simulink model "mainmodel"  (R2020a)
settings: Solver=VariableStepAuto  StartTime=0.0  StopTime=10.0  MaxStep=0.04  RelTol=1e-3
undefined symbols (not defined in the file): Iei, Iv, Rfd, Rw
settings Model: Creator=Bhanu  LastModifiedBy=Bhanu

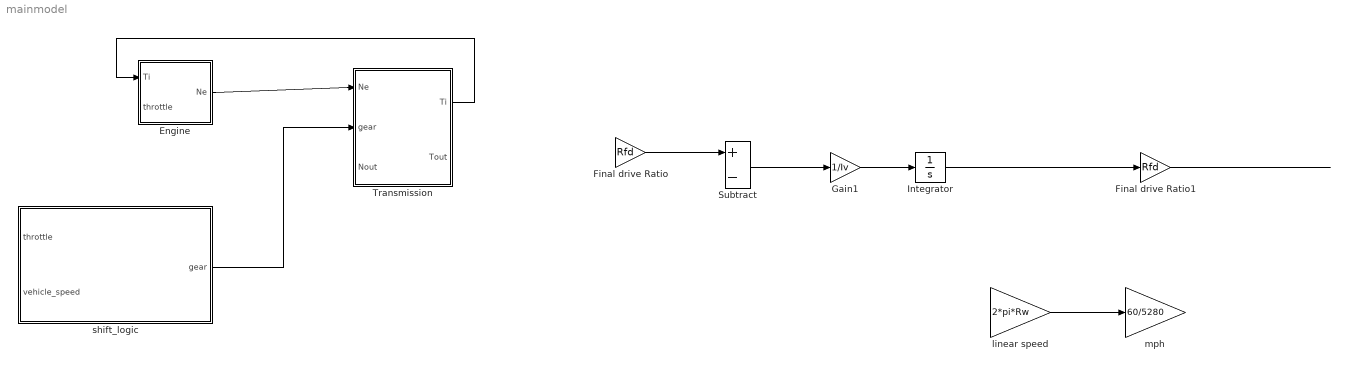
== system mainmodel ==
  "Engine " : Subsystem
  Final drive Ratio : Gain  Gain=Rfd
  Final drive Ratio1 : Gain  Gain=Rfd
  Gain1 : Gain  Gain=1/Iv
  Integrator : Integrator
  Subtract : Sum  Inputs=+-
  "Transmission " : Subsystem
  linear speed : Gain  Gain=2*pi*Rw
  mph : Gain  Gain=60/5280
  shift_logic : Stateflow chart  TreatAsAtomicUnit=on
  wires:
  "Engine "/1(Ne) -> "Transmission "/1(Ne)
  "Transmission "/1(Ti) -> "Engine "/1(Ti)
  shift_logic/1(gear) -> "Transmission "/2(gear)
  Final drive Ratio/1 -> Subtract/1
  Subtract/1 -> Gain1/1
  Gain1/1 -> Integrator/1
  Integrator/1 -> Final drive Ratio1/1
  Final drive Ratio1/1 -> ?
  linear speed/1 -> mph/1

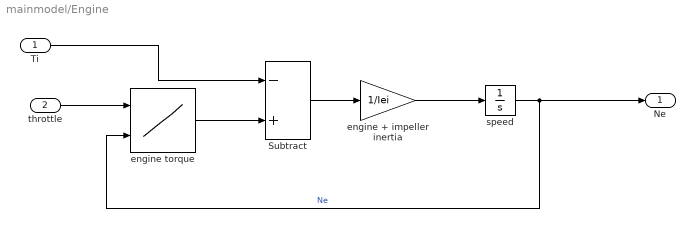
== system mainmodel/Engine  ==
  Ti : Inport
  throttle : Inport  Port=2
  Subtract : Sum  Inputs=-+
  engine + impeller inertia : Gain  Gain=1/Iei
  engine torque : Lookup_n-D  BreakpointsForDimension1=[1:3]  BreakpointsForDimension2=[1:3]  InternalRulePriority=Speed  RndMeth=Simplest  InputSameDT=on
  speed : Integrator  LimitOutput=on  UpperSaturationLimit=5  LowerSaturationLimit=-5
  Ne : Outport
  wires:
  Subtract/1 -> engine + impeller inertia/1
  engine torque/1 -> Subtract/2
  speed/1 -> Ne/1, engine torque/2  "Ne"
  engine + impeller inertia/1 -> speed/1
  Ti/1 -> Subtract/1
  throttle/1 -> engine torque/1

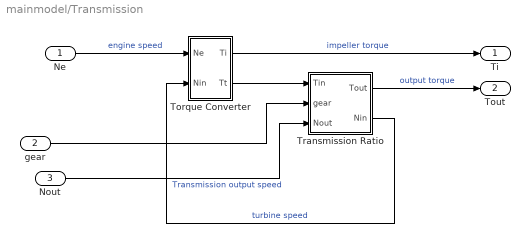
== system mainmodel/Transmission  ==
  Ne : Inport
  gear : Inport  Port=2
  Nout : Inport  Port=3
  Torque Converter : Subsystem
  Transmission Ratio : Subsystem
  Ti : Outport
  Tout : Outport  Port=2
  wires:
  Torque Converter/2(Tt) -> Transmission Ratio/1(Tin)
  Transmission Ratio/2(Nin) -> Torque Converter/2(Nin)  "turbine speed"
  Transmission Ratio/1(Tout) -> Tout/1  "output torque"
  Torque Converter/1(Ti) -> Ti/1  "impeller torque"
  Nout/1 -> Transmission Ratio/3(Nout)  "Transmission output speed"
  Ne/1 -> Torque Converter/1(Ne)  "engine speed"
  gear/1 -> Transmission Ratio/2(gear)

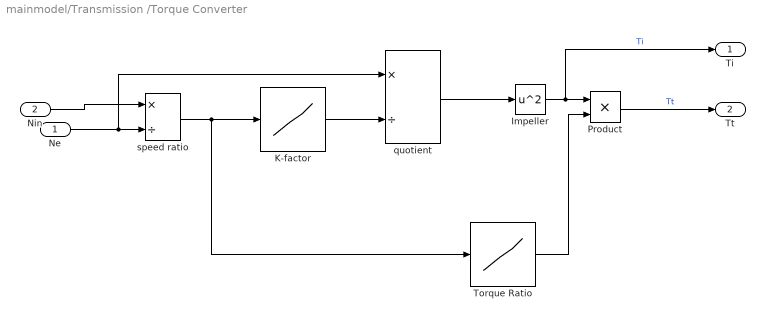
== system mainmodel/Transmission /Torque Converter ==
  Ne : Inport
  Nin : Inport  Port=2
  Impeller : Math  Operator=square  SaturateOnIntegerOverflow=on
  K-factor : Lookup_n-D  NumberOfTableDimensions=1  BreakpointsForDimension1=[-5:5]  Table=tanh([-5:5])  InternalRulePriority=Speed  RndMeth=Simplest  InputSameDT=on
  Product : Product
  Torque Ratio : Lookup_n-D  NumberOfTableDimensions=1  BreakpointsForDimension1=[-5:5]  Table=tanh([-5:5])  InternalRulePriority=Speed  RndMeth=Simplest  InputSameDT=on
  quotient : Product  Inputs=*/
  speed ratio : Product  Inputs=*/
  Ti : Outport
  Tt : Outport  Port=2
  wires:
  speed ratio/1 -> Torque Ratio/1, K-factor/1
  Impeller/1 -> Ti/1, Product/1  "Ti"
  Ne/1 -> quotient/1, speed ratio/2
  Nin/1 -> speed ratio/1
  quotient/1 -> Impeller/1
  K-factor/1 -> quotient/2
  Torque Ratio/1 -> Product/2
  Product/1 -> Tt/1  "Tt"

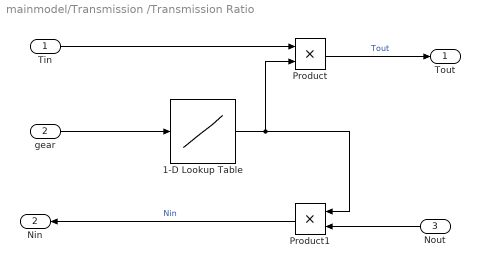
== system mainmodel/Transmission /Transmission Ratio ==
  Tin : Inport
  gear : Inport  Port=2
  Nout : Inport  Port=3
  1-D Lookup Table : Lookup_n-D  NumberOfTableDimensions=1  BreakpointsForDimension1=[-5:5]  Table=tanh([-5:5])  InternalRulePriority=Speed  RndMeth=Simplest  InputSameDT=on
  Product : Product
  Product1 : Product
  Tout : Outport
  Nin : Outport  Port=2
  wires:
  Product/1 -> Tout/1  "Tout"
  1-D Lookup Table/1 -> Product/2, Product1/1
  Product1/1 -> Nin/1  "Nin"
  Tin/1 -> Product/1
  gear/1 -> 1-D Lookup Table/1
  Nout/1 -> Product1/2

== stateflow chart mainmodel/shift_logic ==
  state gear_selection
    state gear_state [parallel]
      settings: executionOrder=2
      state first
        en: gear = 1;
      state second
        en: gear = 2;
      state third
        en: gear = 3;
      state fourth
        en: gear = 4;
      first -> second : UPSHIFT12
      second -> third [order 1] : UPSHIFT23
      third -> fourth [order 1] : UPSHIFT34
      (default) -> first
      second -> first [order 2] : DOWNSHIFT21
      third -> second [order 2] : DOWNSHIFT32
      fourth -> third : DOWNSHIFT43
    state selection_state [parallel]
      during: down_threshold = ml('interp2([1:4],downth, downtab, %g, %g)', gear, throttle);
      up_threshold = ml('interp2([1:4],upth, uptab, %g, %g)', gear, throttle);
      settings: executionOrder=1
      state upshift_confirm1
        en: tdn = t;
      state steady_state
      state upshift_confirm
        en: tup = t;
      (default) -> steady_state
      steady_state -> upshift_confirm1 [order 2] : [vehicle_speed < down_threshold]
      steady_state -> upshift_confirm [order 1] : [vehicle_speed > up_threshold]
      upshift_confirm1 -> (junction 31) [order 2] : [t-tdn >= Tconfirm & vehicle_speed <= down_threshold]
      upshift_confirm1 -> steady_state [order 1] : [vehicle_speed > down_threshold]
      (junction 27) -> steady_state
      (junction 28) -> steady_state
      upshift_confirm -> steady_state [order 1] : [vehicle_speed < up_threshold]
      upshift_confirm -> (junction 32) [order 2] : [t-tup >= Tconfirm & vehicle_speed >= up_threshold]
      (junction 32) -> (junction 28) [order 3] : [gear == 3]/{UPSHIFT34}
      (junction 31) -> (junction 27) [order 3] : [gear == 4]/{DOWNSHIFT43}
      (junction 32) -> (junction 28) [order 2] : [gear == 2]/{UPSHIFT23}
      (junction 31) -> (junction 27) [order 2] : [gear == 3]/{DOWNSHIFT32}
      (junction 32) -> (junction 28) [order 1] : [gear == 1]/{UPSHIFT12}
      (junction 31) -> (junction 27) [order 1] : [gear == 2]/{DOWNSHIFT21}
  (default) -> gear_selection
  data: gear output; throttle input; vehicle_speed input; Tconfirm local; ml local; down_threshold local; tdn local; tup local; up_threshold local
  events: DOWNSHIFT21 local FUNCTION_CALL_EVENT; DOWNSHIFT32 local FUNCTION_CALL_EVENT; DOWNSHIFT43 local FUNCTION_CALL_EVENT; UPSHIFT12 local FUNCTION_CALL_EVENT; UPSHIFT23 local FUNCTION_CALL_EVENT; UPSHIFT34 local FUNCTION_CALL_EVENT
